simulink library "magnetorquer_processing_lib"  (R2016b)
settings: Solver=ode45  StartTime=0.0  StopTime=10.0  RelTol=1e-3  EnableMultiTasking=on
undefined symbols (not defined in the file or in its folder): fsw_params
settings Model: Creator=Taylor  LastModifiedBy=Taylor
settings DataIOCC: LimitDataPoints=on
settings OptimizationCC: LifeSpan=inf
settings DebuggingCC: AllowSymbolicDim=off  SFUnexpectedBacktrackingDiag=warning  SFNoUnconditionalDefaultTransitionDiag=warning  SFExecutionAtInitializationDiag=none
settings GRTTargetCC: TargetLangStandard=C89/C90 (ANSI)  GeneratePreprocessorConditionals=Disable all
settings ConfigComp: CovMetricSettings=dw  CovHtmlReporting=on  CovSaveCumulativeToWorkspaceVar=on  CovSaveSingleToWorkspaceVar=on  CovExternalEMLEnable=off

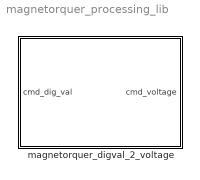
== system magnetorquer_processing_lib ==
  magnetorquer_digval_2_voltage : Subsystem

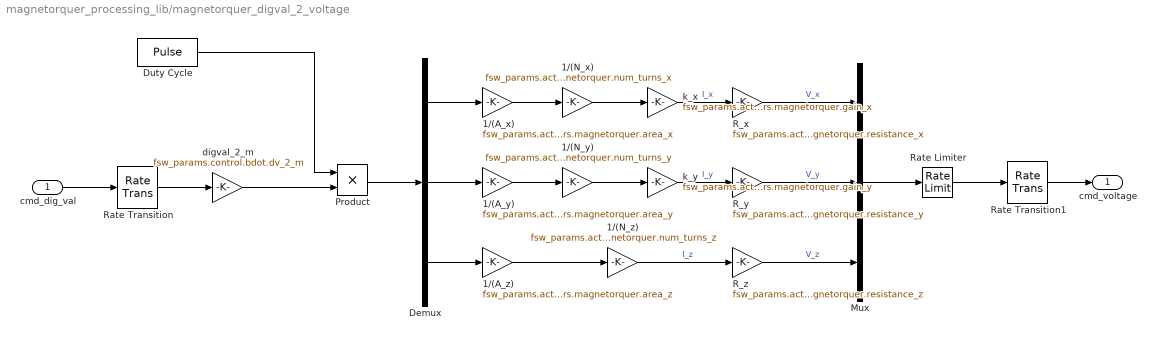
== system magnetorquer_processing_lib/magnetorquer_digval_2_voltage ==
  cmd_dig_val : Inport
  1/(A_x) : Gain  Gain=fsw_params.actuators.magnetorquer.area_x
  1/(A_y) : Gain  Gain=fsw_params.actuators.magnetorquer.area_y
  1/(A_z) : Gain  Gain=fsw_params.actuators.magnetorquer.area_z
  1/(N_x) : Gain  Gain=fsw_params.actuators.magnetorquer.num_turns_x
  1/(N_y) : Gain  Gain=fsw_params.actuators.magnetorquer.num_turns_y
  1/(N_z) : Gain  Gain=fsw_params.actuators.magnetorquer.num_turns_z
  Demux : Demux  Outputs=3
  Duty Cycle : DiscretePulseGenerator  PulseType=Time based  Period=fsw_params.actuators.magnetorquer.duty_cycle_period_s  PulseWidth=fsw_params.actuators.magnetorquer.pct_duty_cycle_on
  Mux : Mux  Inputs=3
  Product : Product
  R_x : Gain  Gain=fsw_params.actuators.magnetorquer.resistance_x
  R_y : Gain  Gain=fsw_params.actuators.magnetorquer.resistance_y
  R_z : Gain  Gain=fsw_params.actuators.magnetorquer.resistance_z
  Rate Limiter : RateLimiter  RisingSlewLimit=fsw_params.actuators.magnetorquer.max_rate  FallingSlewLimit=-fsw_params.actuators.magnetorquer.max_rate  SampleTimeMode=inherited
  Rate Transition : RateTransition  X0=fsw_params.actuators.magnetorquer.ic.rt_in  OutPortSampleTime=fsw_params.actuators.magnetorquer.sample_time_s
  Rate Transition1 : RateTransition  X0=fsw_params.actuators.magnetorquer.ic.rt_out  OutPortSampleTimeOpt=Inherit
  digval_2_m : Gain  Gain=fsw_params.control.bdot.dv_2_m
  k_x : Gain  Gain=fsw_params.actuators.magnetorquer.gain_x
  k_y : Gain  Gain=fsw_params.actuators.magnetorquer.gain_y
  cmd_voltage : Outport
  wires:
  cmd_dig_val/1 -> Rate Transition/1
  Demux/3 -> 1/(A_z)/1
  1/(A_z)/1 -> 1/(N_z)/1
  R_z/1 -> Mux/3  "V_z"
  Demux/2 -> 1/(A_y)/1
  1/(A_y)/1 -> 1/(N_y)/1
  1/(N_y)/1 -> k_y/1
  Demux/1 -> 1/(A_x)/1
  1/(A_x)/1 -> 1/(N_x)/1
  1/(N_x)/1 -> k_x/1
  k_y/1 -> R_y/1  "I_y"
  k_x/1 -> R_x/1  "I_x"
  R_y/1 -> Mux/2  "V_y"
  R_x/1 -> Mux/1  "V_x"
  Mux/1 -> Rate Limiter/1
  Rate Transition/1 -> digval_2_m/1
  Rate Transition1/1 -> cmd_voltage/1
  1/(N_z)/1 -> R_z/1  "I_z"
  Product/1 -> Demux/1
  digval_2_m/1 -> Product/2
  Duty Cycle/1 -> Product/1
  Rate Limiter/1 -> Rate Transition1/1
